simulink model "Model_I92_Landing_NL"  (Simulink 6.6)
settings: Solver=ode45  StartTime=tmin  StopTime=tmax  MaxStep=dt  RelTol=1e-3
values from neighbouring files (symbols this model uses):
  dt = 0.01    [Pgm_G11_Superposition.m]    (also in Pgm_G12_Num_Integration.m; Pgm_G13_Frequency_Domain.m = 0.0625; Pgm_H2_Response_Gusts_Control.m = 0.001; Pgm_H3_Ase_Gusts_Pid.m = 0.001)
  kt = 1000e3    (= 1000000)    [Pgm_I92_Landing.m]
  m = [m1 m2 m3 -m4; m2 m5 m4 -m6; m3 m4 m1 -m2; -m4 -m6 -m2 m5]    [Pgm_G3_FE_Solution.m]    (also in Pgm_H2_Response_Gusts_Control.m = 100; Pgm_H3_Ase_Gusts_Pid.m = 100; Pgm_I1_Rigid_Aircraft_Data.m = 10000; Prg_H1_Calcs.m = 100)
  mt = 100    [Pgm_I92_Landing.m]
  W_e = 0    [Pgm_I6_Dynamic_Manoeuvres.m]    (also in Pgm_I92_Landing.m = 3)
  z = kappa * s - theta * c/2    [Pgm_H3_Ase_Gusts_Pid.m]    (also in Pgm_I92_Landing.m = [0: dz: zS];  [dummy, nz] = size(z))
  zdot = [-1.5: 0.005: 3];  [dummy, nzdot] = size(zdot)    [Pgm_I92_Landing.m]
undefined symbols (not defined in the file or in its folder): Fd, Fdamp
settings Model: Creator=Jan Wright  LastModifiedBy=Jan Wright
settings DataIOCC: InitialState=z_Mdot=W_e  SaveOutput=off  SaveTime=off  SignalLoggingName=sigsOut
settings DebuggingCC: SignalResolutionControl=TryResolveAllWithWarning  SolverPrmCheckMsg=none  MultiTaskDSMMsg=warning  MultiTaskCondExecSysMsg=none  StrictBusMsg=None
settings HardwareCC: TargetUnknown=on
settings RTWCC: IncludeERTFirstTime=on
settings GRTTargetCC: ModelReferenceCompliant=off  MatFileLogging=off

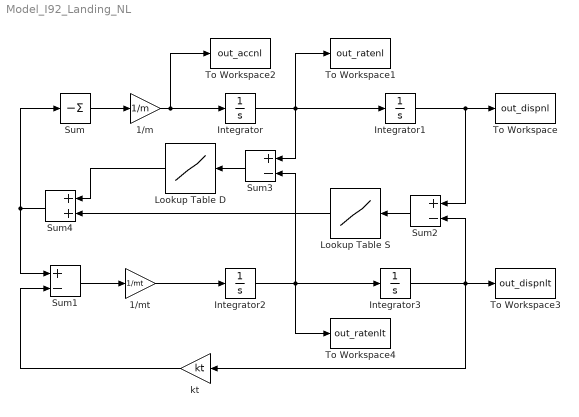
== system Model_I92_Landing_NL ==
  1/m : Gain  Gain=1/m  SaturateOnIntegerOverflow=on
  1/mt : Gain  Gain=1/mt  SaturateOnIntegerOverflow=on
  Integrator : Integrator  InitialCondition=W_e
  Integrator1 : Integrator
  Integrator2 : Integrator  InitialCondition=W_e
  Integrator3 : Integrator
  Lookup Table D : Lookup  Orientation=left  InputValues=zdot  OutputValues=Fdamp
  Lookup Table S : Lookup  Orientation=left  InputValues=z  OutputValues=Fd
  Sum : Sum  Inputs=-  SaturateOnIntegerOverflow=on
  Sum1 : Sum  Inputs=+-  SaturateOnIntegerOverflow=on
  Sum2 : Sum  Orientation=left  Inputs=+-  SaturateOnIntegerOverflow=on
  Sum3 : Sum  Orientation=left  Inputs=+-  SaturateOnIntegerOverflow=on
  Sum4 : Sum  Orientation=left  SaturateOnIntegerOverflow=on
  To Workspace : ToWorkspace  VariableName=out_dispnl  SampleTime=dt  SaveFormat=Array
  To Workspace1 : ToWorkspace  VariableName=out_ratenl  SampleTime=dt  SaveFormat=Array
  To Workspace2 : ToWorkspace  VariableName=out_accnl  SampleTime=dt  SaveFormat=Array
  To Workspace3 : ToWorkspace  VariableName=out_dispnlt  SampleTime=dt  SaveFormat=Array
  To Workspace4 : ToWorkspace  VariableName=out_ratenlt  SampleTime=dt  SaveFormat=Array
  kt : Gain  Orientation=left  Gain=kt  SaturateOnIntegerOverflow=on
  wires:
  Integrator/1 -> To Workspace1/1, Integrator1/1, Sum3/1
  Integrator1/1 -> To Workspace/1, Sum2/1
  Sum/1 -> 1/m/1
  1/m/1 -> Integrator/1, To Workspace2/1
  1/mt/1 -> Integrator2/1
  Integrator2/1 -> Integrator3/1, To Workspace4/1, Sum3/2
  Sum1/1 -> 1/mt/1
  Integrator3/1 -> kt/1, To Workspace3/1, Sum2/2
  kt/1 -> Sum1/2
  Sum2/1 -> Lookup Table S/1
  Sum3/1 -> Lookup Table D/1
  Lookup Table D/1 -> Sum4/1
  Lookup Table S/1 -> Sum4/2
  Sum4/1 -> Sum1/1, Sum/1
